simulink model "Shoulder_closeloop1"  (Simulink 6.4)
settings: Solver=FixedStepDiscrete  StartTime=0.0  StopTime=inf  FixedStep=0.001  RelTol=1e-3
undefined symbols (not defined in the file): REAL, TIME
libraries: simulink x12, xpclib x2, RT x1
settings Model: LastModifiedBy=Maggia

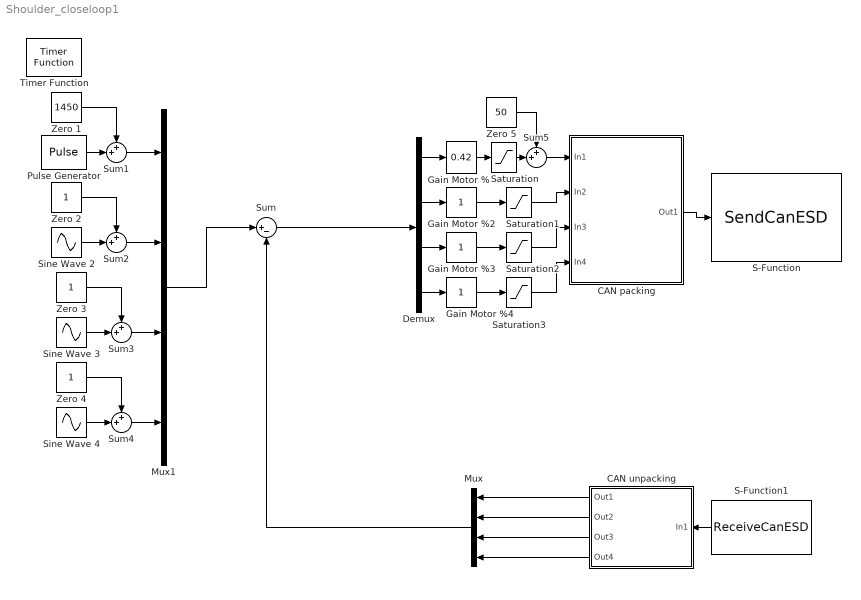
== system Shoulder_closeloop1 ==
  CAN packing : Subsystem
  CAN unpacking : Subsystem  Orientation=left
  Demux : Demux
  Gain Motor %1 : simulink/Math Operations/Slider Gain  SystemSampleTime=-1  low=0  gain=0.42  high=2
  Gain Motor %2 : simulink/Math Operations/Slider Gain  SystemSampleTime=-1  low=0  gain=1  high=100
  Gain Motor %3 : simulink/Math Operations/Slider Gain  SystemSampleTime=-1  low=0  gain=1  high=100
  Gain Motor %4 : simulink/Math Operations/Slider Gain  SystemSampleTime=-1  low=0  gain=1  high=100
  Mux : Mux  Orientation=left
  Mux1 : Mux
  Pulse Generator : DiscretePulseGenerator  PulseType=Time based  Amplitude=300  Period=3  PulseWidth=50
  S-Function : S-Function  FunctionName=SendCanESD  Parameters=(baudrate-1),msgid,length  mask{baudrate=1000 Kbits/s, msgid=15, length=8}
      mask prompts: msgid "Message ID"; length "Message Length"
      mask StyleString: popup(1000 Kbits/s|500  Kbits/s),edit,edit
      mask Display:
      | fprintf('SEND CAN\n')
      | fprintf('\nID %d',msgid);
      | port_label('input',1,'message');
      | color('red');port_label('output',1,'status');
  S-Function1 : S-Function  Orientation=left  FunctionName=ReceiveCanESD  Parameters=msgID  mask{msgID=16}
      mask prompts: msgID "Message ID"
      mask Display:
      | fprintf('RECEIVE CAN\n')
      | fprintf('\nID %d',msgID);
      | port_label('output',1,'data');
  Saturation{,1..3} (4 alike) : Saturate  UpperLimit=50  LowerLimit=-50
  Sine Wave 2 : Sin  Amplitude=0  SampleTime=0
  Sine Wave 3 : Sin  Amplitude=0  SampleTime=0
  Sine Wave 4 : Sin  Amplitude=0  SampleTime=0
  Sum : Sum  Inputs=|+-
  Sum{1..5} (5 alike) : Sum  Inputs=++|
  Timer Function : RT/Timer Function  Priority=287053392  step=1  priority=REAL-TIME  ThPriority=HIGHEST
  Zero 1 : Constant  Value=1450  OutDataType=sfix(16)  ConRadixGroup=Use specified scaling  OutScaling=2^0  SampleTime=inf  FramePeriod=inf
  Zero 2 : Constant  Value=1  OutDataType=sfix(16)  ConRadixGroup=Use specified scaling  OutScaling=2^0  SampleTime=inf  FramePeriod=inf
  Zero 3 : Constant  Value=1  OutDataType=sfix(16)  ConRadixGroup=Use specified scaling  OutScaling=2^0  SampleTime=inf  FramePeriod=inf
  Zero 4 : Constant  Value=1  OutDataType=sfix(16)  ConRadixGroup=Use specified scaling  OutScaling=2^0  SampleTime=inf  FramePeriod=inf
  Zero 5 : Constant  Value=50  OutDataType=sfix(16)  ConRadixGroup=Use specified scaling  OutScaling=2^0  SampleTime=inf  FramePeriod=inf
  wires:
  Gain Motor %1/1 -> Saturation/1
  CAN packing/1(Out1) -> S-Function/1
  S-Function1/1 -> CAN unpacking/1(In1)
  Gain Motor %2/1 -> Saturation1/1
  Gain Motor %3/1 -> Saturation2/1
  Gain Motor %4/1 -> Saturation3/1
  CAN unpacking/1(Out1) -> Mux/1
  CAN unpacking/2(Out2) -> Mux/2
  CAN unpacking/3(Out3) -> Mux/3
  CAN unpacking/4(Out4) -> Mux/4
  Mux/1 -> Sum/2
  Demux/1 -> Gain Motor %1/1
  Demux/2 -> Gain Motor %2/1
  Demux/3 -> Gain Motor %3/1
  Demux/4 -> Gain Motor %4/1
  Sum/1 -> Demux/1
  Pulse Generator/1 -> Sum1/2
  Zero 1/1 -> Sum1/1
  Sum1/1 -> Mux1/1
  Sine Wave 2/1 -> Sum2/2
  Zero 2/1 -> Sum2/1
  Sum2/1 -> Mux1/2
  Sine Wave 3/1 -> Sum3/2
  Zero 3/1 -> Sum3/1
  Sum3/1 -> Mux1/3
  Sine Wave 4/1 -> Sum4/2
  Zero 4/1 -> Sum4/1
  Sum4/1 -> Mux1/4
  Mux1/1 -> Sum/1
  Saturation/1 -> Sum5/2
  Saturation1/1 -> CAN packing/2(In2)
  Saturation2/1 -> CAN packing/3(In3)
  Saturation3/1 -> CAN packing/4(In4)
  Zero 5/1 -> Sum5/1
  Sum5/1 -> CAN packing/1(In1)

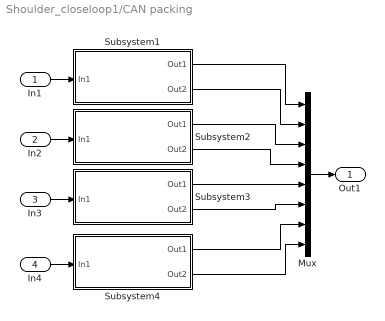
== system Shoulder_closeloop1/CAN packing ==
  In1 : Inport
  In2 : Inport  Port=2
  In3 : Inport  Port=3
  In4 : Inport  Port=4
  Mux : Mux  Inputs=8
  Subsystem1 : Subsystem
  Subsystem2 : Subsystem
  Subsystem3 : Subsystem
  Subsystem4 : Subsystem
  Out1 : Outport
  wires:
  Subsystem1/1(Out1) -> Mux/1
  Subsystem1/2(Out2) -> Mux/2
  Subsystem2/1(Out1) -> Mux/3
  Subsystem2/2(Out2) -> Mux/4
  Subsystem3/1(Out1) -> Mux/5
  Subsystem3/2(Out2) -> Mux/6
  Subsystem4/1(Out1) -> Mux/7
  Subsystem4/2(Out2) -> Mux/8
  In1/1 -> Subsystem1/1(In1)
  In2/1 -> Subsystem2/1(In1)
  Mux/1 -> Out1/1
  In3/1 -> Subsystem3/1(In1)
  In4/1 -> Subsystem4/1(In1)

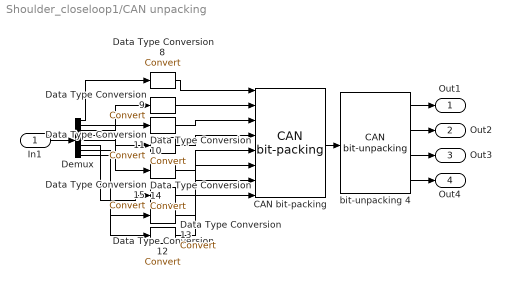
== system Shoulder_closeloop1/CAN unpacking ==
  In1 : Inport
  " bit-unpacking 4" : xpclib/CAN/Utilities/CAN bit-unpacking   bitpatterns={ [0:15] [16:31] [32:47] [48:63]}  dtypes={ 'uint16' 'uint16' 'uint16' 'uint16'}
  "CAN bit-packing " : xpclib/CAN/Utilities/CAN bit-packing   bitpatterns={ [0:7] [8:15] [16:23] [24:31] [32:39] [40:47] [48:55] [56:63] }
  Data Type Conversion{8..15} (8 alike) : DataTypeConversion  OutDataTypeMode=uint8
  Demux : Demux  Outputs=8
  Out1 : Outport
  Out2 : Outport  Port=2
  Out3 : Outport  Port=3
  Out4 : Outport  Port=4
  wires:
  "CAN bit-packing "/1 -> " bit-unpacking 4"/1
  Data Type Conversion8/1 -> "CAN bit-packing "/1
  Data Type Conversion9/1 -> "CAN bit-packing "/2
  Data Type Conversion10/1 -> "CAN bit-packing "/3
  Data Type Conversion11/1 -> "CAN bit-packing "/4
  Data Type Conversion14/1 -> "CAN bit-packing "/5
  Data Type Conversion15/1 -> "CAN bit-packing "/6
  Data Type Conversion12/1 -> "CAN bit-packing "/7
  Data Type Conversion13/1 -> "CAN bit-packing "/8
  Demux/1 -> Data Type Conversion8/1
  Demux/2 -> Data Type Conversion9/1
  Demux/3 -> Data Type Conversion10/1
  Demux/4 -> Data Type Conversion11/1
  Demux/5 -> Data Type Conversion14/1
  Demux/6 -> Data Type Conversion15/1
  Demux/7 -> Data Type Conversion12/1
  Demux/8 -> Data Type Conversion13/1
  " bit-unpacking 4"/1 -> Out1/1
  " bit-unpacking 4"/2 -> Out2/1
  In1/1 -> Demux/1
  " bit-unpacking 4"/3 -> Out3/1
  " bit-unpacking 4"/4 -> Out4/1

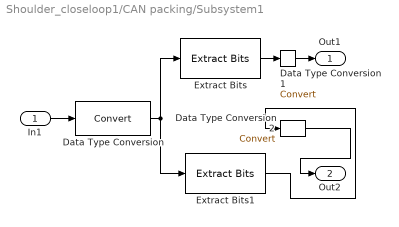
== system Shoulder_closeloop1/CAN packing/Subsystem1 ==
  In1 : Inport
  Data Type Conversion : DataTypeConversion  OutDataTypeMode=uint16
  Data Type Conversion1 : DataTypeConversion  OutDataTypeMode=double
  Data Type Conversion2 : DataTypeConversion  OutDataTypeMode=double
  Extract Bits : simulink/Logic and Bit Operations/Extract Bits  SystemSampleTime=-1  bitsToExtract=Range of bits  numBits=8  bitIdxRange=[0 7]  outScalingMode=Treat bit field as an integer
  Extract Bits1 : simulink/Logic and Bit Operations/Extract Bits  SystemSampleTime=-1  bitsToExtract=Range of bits  numBits=8  bitIdxRange=[8 15]  outScalingMode=Treat bit field as an integer
  Out1 : Outport
  Out2 : Outport  Port=2
  wires:
  Data Type Conversion/1 -> Extract Bits1/1, Extract Bits/1
  Extract Bits/1 -> Data Type Conversion1/1
  In1/1 -> Data Type Conversion/1
  Data Type Conversion1/1 -> Out1/1
  Data Type Conversion2/1 -> Out2/1
  Extract Bits1/1 -> Data Type Conversion2/1

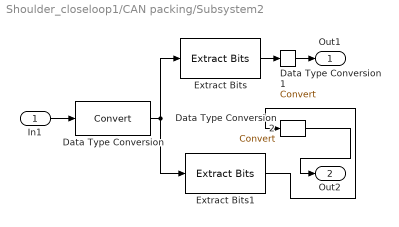
== system Shoulder_closeloop1/CAN packing/Subsystem2 ==
  In1 : Inport
  Data Type Conversion : DataTypeConversion  OutDataTypeMode=uint16
  Data Type Conversion1 : DataTypeConversion  OutDataTypeMode=double
  Data Type Conversion2 : DataTypeConversion  OutDataTypeMode=double
  Extract Bits : simulink/Logic and Bit Operations/Extract Bits  SystemSampleTime=-1  bitsToExtract=Range of bits  numBits=8  bitIdxRange=[0 7]  outScalingMode=Treat bit field as an integer
  Extract Bits1 : simulink/Logic and Bit Operations/Extract Bits  SystemSampleTime=-1  bitsToExtract=Range of bits  numBits=8  bitIdxRange=[8 15]  outScalingMode=Treat bit field as an integer
  Out1 : Outport
  Out2 : Outport  Port=2
  wires:
  Data Type Conversion/1 -> Extract Bits1/1, Extract Bits/1
  Extract Bits/1 -> Data Type Conversion1/1
  In1/1 -> Data Type Conversion/1
  Data Type Conversion1/1 -> Out1/1
  Data Type Conversion2/1 -> Out2/1
  Extract Bits1/1 -> Data Type Conversion2/1

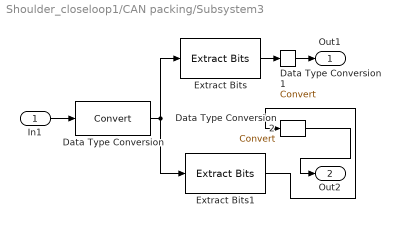
== system Shoulder_closeloop1/CAN packing/Subsystem3 ==
  In1 : Inport
  Data Type Conversion : DataTypeConversion  OutDataTypeMode=uint16
  Data Type Conversion1 : DataTypeConversion  OutDataTypeMode=double
  Data Type Conversion2 : DataTypeConversion  OutDataTypeMode=double
  Extract Bits : simulink/Logic and Bit Operations/Extract Bits  SystemSampleTime=-1  bitsToExtract=Range of bits  numBits=8  bitIdxRange=[0 7]  outScalingMode=Treat bit field as an integer
  Extract Bits1 : simulink/Logic and Bit Operations/Extract Bits  SystemSampleTime=-1  bitsToExtract=Range of bits  numBits=8  bitIdxRange=[8 15]  outScalingMode=Treat bit field as an integer
  Out1 : Outport
  Out2 : Outport  Port=2
  wires:
  Data Type Conversion/1 -> Extract Bits1/1, Extract Bits/1
  Extract Bits/1 -> Data Type Conversion1/1
  In1/1 -> Data Type Conversion/1
  Data Type Conversion1/1 -> Out1/1
  Data Type Conversion2/1 -> Out2/1
  Extract Bits1/1 -> Data Type Conversion2/1

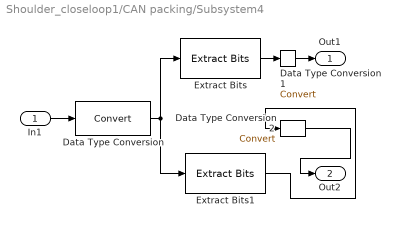
== system Shoulder_closeloop1/CAN packing/Subsystem4 ==
  In1 : Inport
  Data Type Conversion : DataTypeConversion  OutDataTypeMode=uint16
  Data Type Conversion1 : DataTypeConversion  OutDataTypeMode=double
  Data Type Conversion2 : DataTypeConversion  OutDataTypeMode=double
  Extract Bits : simulink/Logic and Bit Operations/Extract Bits  SystemSampleTime=-1  bitsToExtract=Range of bits  numBits=8  bitIdxRange=[0 7]  outScalingMode=Treat bit field as an integer
  Extract Bits1 : simulink/Logic and Bit Operations/Extract Bits  SystemSampleTime=-1  bitsToExtract=Range of bits  numBits=8  bitIdxRange=[8 15]  outScalingMode=Treat bit field as an integer
  Out1 : Outport
  Out2 : Outport  Port=2
  wires:
  Data Type Conversion/1 -> Extract Bits1/1, Extract Bits/1
  Extract Bits/1 -> Data Type Conversion1/1
  In1/1 -> Data Type Conversion/1
  Data Type Conversion1/1 -> Out1/1
  Data Type Conversion2/1 -> Out2/1
  Extract Bits1/1 -> Data Type Conversion2/1
